simulink model "dSpaceModel_2"  (R2023a)
settings: Solver=ode1  StartTime=0.0  StopTime=inf  FixedStep=0.001  RelTol=1e-3
PostLoadFcn:
  | , if any(exist('dsrtsu_mdlpostloadfcn', 'file') ~= 0), dsrtsu_mdlpostloadfcn('Execute', bdroot); end,
InitFcn:
  | , if any(exist('rtifpga_mdlclblib', 'file') ~= 0), rtifpga_mdlclblib('Init', bdroot); end,
model workspace (MAT data in the model file):
  mode = 2
libraries: rti1202serlib x5, simulink x2, svdutilitieslib x1
(part 1 of 3)
Description:
  | Standard RTI1202 template.
  | Supported MATLAB version:  R2023a.
settings Model: Tag=RTI1202  DSRTSU_INTERNAL_RTI_VER=620  DSRTSU_INTERNAL_RTI_TYPE=rti1202  RTICANMMDATA=struct('GeneralSetupData',struct('modelroot','C:\Users\VM-User\Desktop\MigrationScripts','generalsettings',struct('filesettings',struct('destfolder',struct('Name','RTICANMM_FILES','Check',1),'buildfolder',struct('Name','.','Check',1),'AbsDestfolder',struct('Name','C:\Users\VM-User\Desktop\MigrationScripts\RTICANMM_FILES'),'AbsBuildfolder',struct('Name','C:\Users\VM-User\Desktop\MigrationScripts'))),'options',struct('addpaths',1,'rmpaths',1,'addtrcexclusion',true,'cannavigator',struct('checkmonitoring',0),'show_usrtrc',0,'use_usrtrc',0),'advanced',struct('options',ones(1,100)),'MPSetup',{{}},'RTI',struct('Type','RTI1202','Ver','7.17','Date','02-Nov-2021'),'modelname','','block','untitled'))  DSRTSU_INTERNAL_RTIFPGA=200  DSRTSU_INTERNAL_RTISTBM_VER=23.1  Creator=yd12yqyf  LastModifiedBy=ej62ixyv
settings SolverCC: AlgebraicLoopSolver=TrustRegion
settings DataIOCC: ReturnWorkspaceOutputs=off
settings OptimizationCC: BlockReduction=off  OptimizeBlockIOStorage=off  BufferReuse=off  ReuseModelBlockBuffer=off  GlobalBufferReuse=off  ExpressionFolding=off  LocalBlockOutputs=off  OptimizeDataStoreBuffers=off  BusAssignmentInplaceUpdate=off
settings DebuggingCC: UnderSpecifiedDataTypeMsg=warning  UnconnectedInputMsg=warning  UnconnectedOutputMsg=warning  UnconnectedLineMsg=warning  PregeneratedLibrarySubsystemCodeDiagnostic=none  UnderSpecifiedDimensionMsg=warning  ArithmeticOperatorsInVariantConditions=warning
settings HardwareCC: ProdBitPerPointer=32  ProdBitPerSizeT=32  ProdBitPerPtrDiffT=32  ProdLargestAtomicInteger=Integer  ProdEndianess=BigEndian  ProdWordSize=32  ProdLongLongMode=on  ProdHWDeviceType=Custom Processor->Custom  TargetIntDivRoundTo=Zero  TargetEndianess=BigEndian  TargetHWDeviceType=Custom Processor->Custom
settings ModelReferenceCC: EnableRefExpFcnMdlSchedulingChecks=on  EnableParallelModelReferenceBuilds=on  ParallelModelReferenceMATLABWorkerInit=Load Top Model
settings SFSimCC: SimUseLocalCustomCode=off  MATLABDynamicMemAlloc=off  CustomCodeUndefinedFunction=UseInterfaceOnly
settings RTWCC: Description=dSPACE DS1202 Hardware Platform  SystemTargetFile=rti1202.tlc  MakeCommand=make_rti  TemplateMakefile=rti1202.tmf  RTWUseLocalCustomCode=off  DLArmComputeVersion=19.05
settings CodeAppCC: StateflowObjectComments=on
settings STFCustomTargetCC: ParMdlRefBuildCompliant=on  ConcurrentExecutionCompliant=off  GRTInterface=off  UseToolchainInfoCompliant=off  SystemTargetFile=rti1202.tlc
settings GRTTargetCC: CompOptLevelCompliant=off  ConcurrentExecutionCompliant=off  CombineOutputUpdateFcns=off  MatFileLogging=off  CPPClassGenCompliant=off  UseToolchainInfoCompliant=off
settings ConfigComp: CovMetricSettings=dswe

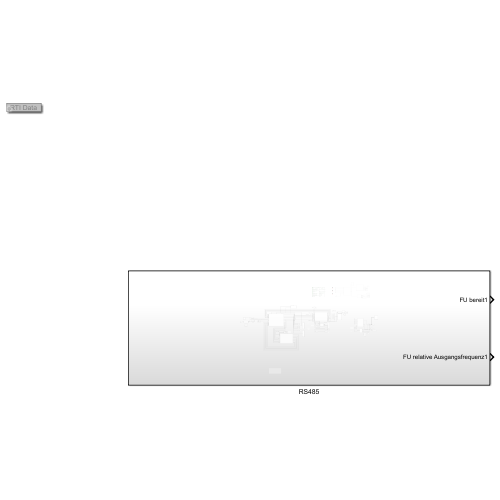
[thumbnail: Simulink's stored preview of the top-level diagram]
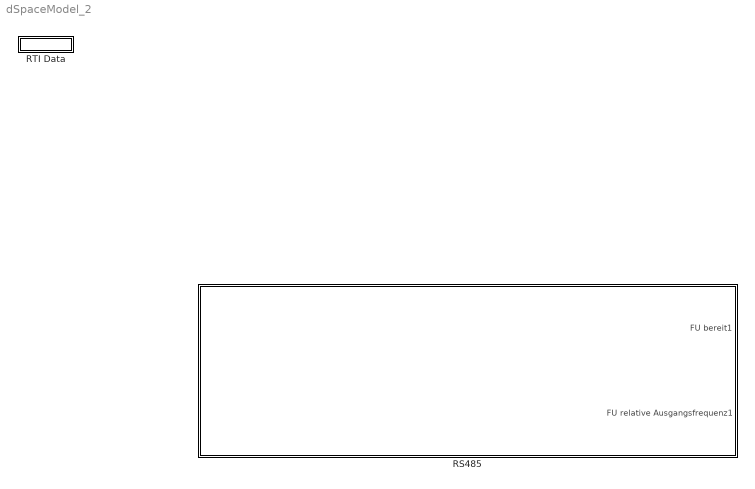
== system dSpaceModel_2 ==
  RS485 : Subsystem
  RTI Data : Subsystem  Tag=struct('RTIDataServer',struct('RTIDataServerVs','2','RTIModelDescription','struct(''main'',''dSpaceModel_2'',''sub'',''dSpaceModel_2'',''isMp'',0)'))  LoadFcn="if exist('rtidc'), try,  rtidc('DataHostBlockClbLoad', gcbh); catch, disp(['Warning: ''LoadFcn'' for RTI Data block failed: ' lasterr]); end, end,"  mask(RTI_DATA_HOST){}
      mask help:
      | RTI Data Block.
      | This block is used by RTI to store internal model-dependent data.
      | Please keep this block on the root level of the model. Deleting this block will result in data loss.
      |
      | NEVER DELETE OR COPY THIS BLOCK!
      settings: CopyFcn="if exist('rtidc'), try,  rtidc('DataHostBlockClbCopy', gcbh); catch, disp(['Warning: ''CopyFcn'' for RTI Data block failed: ' lasterr]); end, end,"  DeleteFcn="if exist('rtidc'), try,  rtidc('DataHostBlockClbDelete', gcbh); catch, disp(['Warning: ''DeleteFcn'' for RTI Data block failed: ' lasterr]); end, end,"  ModelCloseFcn="if exist('rtidc'), try,  rtidc('DataHostBlockClbModelClose', gcbh); catch, disp(['Warning: ''ModelCloseFcn'' for RTI Data block failed: ' lasterr]); end, end,"  PreSaveFcn="if exist('rtidc'), try,  rtidc('DataHostBlockClbPreSave', gcbh); catch, disp(['Warning: ''PreSaveFcn'' for RTI Data block failed: ' lasterr]); end, end,"  PostSaveFcn="if exist('rtidc'), try,  rtidc('DataHostBlockClbPostSave', gcbh); catch, disp(['Warning: ''PostSaveFcn'' for RTI Data block failed: ' lasterr]); end, end,"  NameChangeFcn="if exist('rtidc'), try,  rtidc('DataHostBlockClbNameChange', gcbh); catch, disp(['Warning: ''NameChangeFcn'' for RTI Data block failed: ' lasterr]); end, end,"
      mask Help:
      | RTI Data Block.
      | This block is used by RTI to store internal model-dependent data.
      | Please keep this block on the root level of the model. Deleting this block will result in data loss.
      | 
      | NEVER DELETE OR COPY THIS BLOCK!
      mask Display:
      | text(0.5, 0.5, 'RTI Data', 'HorizontalAlignment', 'center');
      | plot([1 0]);

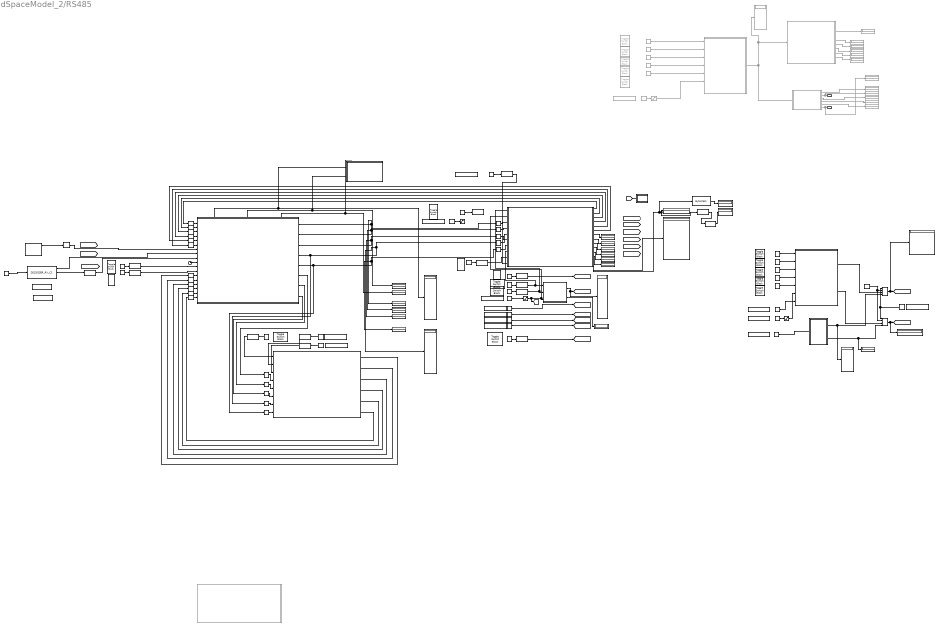
== system dSpaceModel_2/RS485 ==
  note: RX_Data
  note: THRE
  note: %| Bit| Bit value = 0 | Bit value = 1 |
      | %|----|--------------------------------------|------------------------------------|
      | %| 00 | selection between the four "3-10 Preset reference [0]...[3]" |
      | %| 01 | --""-- |
      | %|----|--------------------------------------|------------------------------------|
      | %| 02 | DC brake and stop | performs ramp |
      | %|----|--------------------------------------|------------------------------------|
      | %| 03 | lets the motor coast | starts the motor if conditions are met |
      | %|----|--------------------------------------|------------------------------------|
      | %| 04 | motor speed decreases until stop | |
      | %|----|--------------------------------------|------------------------------------|
      | %| 05 | current output frequency is stored | |
      | %|----|--------------------------------------|------------------------------------|
      | %| 06 | stop using ramp time | starts the motor if conditions are met |
      | %|----|--------------------------------------|------------------------------------|
      | %| 07 | no reset | reset |
      | %|----|--------------------------------------|------------------------------------|
      | %| 08 | | output frequency "3-19 Jog [RPM]" |
      | %|----|--------------------------------------|------------------------------------|
      | %| 09 | ramp 1 active ("3-41" and "3-42") | ramp 2 active ("3-51" and "3-52") |
      | %|----|--------------------------------------|------------------------------------|
      | %| 10 | control word is ignored | control word is used |
      | %|----|--------------------------------------|------------------------------------|
      | %| 11 | relay 01 not activated | relay 01 activated |
      | %|----|--------------------------------------|------------------------------------|
      | %| 12 | relay 04 not activated | relay 04 activated |
      | %|----|--------------------------------------|------------------------------------|
      | %| 13 | parameter set selection "0-10" and "8-55" |
      | %| 14 | |
      | %|----|--------------------------------------|------------------------------------|
      | %| 15 | no reversal | reversal |
  note: expect_len_ZKDM
  note: expect_crc_kind_ZKDM
  note: expect_addr_ZKDM
  note: req_len
  note: req_bytes
  note: req_valid
  note: resp_len
  note: resp_data
  note: resp_err_ZKDM
  note: resp_ok_ZKDM
  note: grant_ZKDM
  note: tx data
  note: tx len
  note: tx trigger
  note: temperature
  Active : Constant  Value=0
  BUS MASTER FSM : Stateflow chart  TreatAsAtomicUnit=on
      settings: PortSchema="{\"entries\":[{\"content\":{\"sides\":[{\"content\":{\"connectorIds\":[\"In4\",\"In16\",\"In18\",\"In8\",\"In14\",\"In10\",\"In1\",\"In2\",\"In3\",\"In6\",\"In11\",\"In12\",\"In5\",\"In15\",\"In17\",\"In7\",\"In13\",\"In9\"]},\"type\":\"ConnectorPlacement.EquallySpacedRectSide\",\"uuid\":\"833d115e-8081-4cb1-98c4-083d374565ad\"},{\"content\":{\"connectorIds\":[\"Out4\",\"Out6\",\"Out5\",\"Out7\",\"Out9\",\"Out10\",\"Out11\",\"Out8\"],\"side\":\"RIGHT\"},\"type\":\"ConnectorPlacement.EquallySpacedRectSide\",\"uuid\":\"f0cbf871-5cea-4f22-8059-874c69130aa3\"},{\"content\":{\"connectorIds\":[\"Out1\",\"Out2\",\"Out3\"],\"side\":\"TOP\"},\"type\":\"ConnectorPlacement.EquallySpacedRectSide\",\"uuid\":\"9def79f2-ef8f-4b80-a903-98ac734b5ab3\"}]},\"type\":\"ConnectorPlacement.EquallySpacedConnector\",\"uuid\":\"db046b19-190e-410f-b654-5051c870f3be\"}],\"packageUris\":[\"http://schema.mathworks.com/mf0/Connector/R2020b\"],\"version\":\"1.0\"}"
  Begrenzung Arbeitstemperatur1 : Saturate  UpperLimit=100  LowerLimit=0  OutDataTypeStr=uint8
  Begrenzung Arbeitstemperatur2 : Saturate  Commented=on  UpperLimit=100  LowerLimit=0
  Begrenzung Arbeitstemperatur3 : Saturate  UpperLimit=100  LowerLimit=0
  Bit Index 6: Transmitter holding register empty (THRE) indicator1 : Selector  InputPortWidth=8  IndexOptions=Starting index (dialog)  Indices=[6]  OutputSizes=1
  Byte Pack : svdutilitieslib/Byte Pack  maskPackedDataType=uint16  datatypes={'uint8'}  byteAlign=1  blockPlatform=tic2000
      settings: LibrarySourceBlock=c2000lib/Target Communication/Byte Pack
  Cast : DataTypeConversion  OutDataTypeStr=uint8  SaturateOnIntegerOverflow=off  RndMeth=Floor
  Cast To Boolean{,1..7,9} (9 alike) : DataTypeConversion  OutDataTypeStr=boolean  SaturateOnIntegerOverflow=off  RndMeth=Floor
  Cast To Boolean10 : DataTypeConversion  OutDataTypeStr=double  SaturateOnIntegerOverflow=off  RndMeth=Floor
  Cast To Boolean11 : DataTypeConversion  OutDataTypeStr=uint8  SaturateOnIntegerOverflow=off  RndMeth=Floor
  Cast To Boolean8 : DataTypeConversion  OutDataTypeStr=double  SaturateOnIntegerOverflow=off  RndMeth=Floor
  Cast To Double : DataTypeConversion  OutDataTypeStr=double  SaturateOnIntegerOverflow=off  RndMeth=Floor
  Cast1 : DataTypeConversion  OutDataTypeStr=uint16  SaturateOnIntegerOverflow=off  RndMeth=Floor
  Clock : Clock
  Constant : Constant  Value=0
  Constant1 : Constant
  Constant10 : Constant
  Constant11 : Constant  Value=34
  Constant12 : Constant  Value=8  OutDataTypeStr=double
  Constant13 : Constant  Value=125
  Constant15 : Constant  Value=0  OutDataTypeStr=uint8
  Constant16 : Constant  Value=0
  Constant19 : Constant  Value=8  OutDataTypeStr=uint32
  Constant2 : Constant  Commented=on  Value=34
  Constant5 : Constant  Value=0
  Constant6 : Constant  Value=12  OutDataTypeStr=uint8
  Constant7 : Constant  Value=31  OutDataTypeStr=uint8
  Constant8 : Constant  Value=8  OutDataTypeStr=uint8
  ConstantSwitch{1,3..6} (5 alike) : Constant  Commented=on
  ConstantSwitch{2,8..11,14} (6 alike) : Constant  Value=0
  ConstantSwitch12 : Constant  Value=34
  ConstantSwitch13 : Constant  Value=10
  ConstantSwitch7 : Constant
  Create 8-Bytes Command : MATLAB Function  TreatAsAtomicUnit=on
  DS1202SER_RX_C2 : rti1202serlib/DS1202SER_RX_C1  Reserved1=[]  Reserved2=[]  Reserved3=[]  Reserved4=[]  DSProperties=struct('RTI',struct('IOBoardType',{{'DS1202','SER'}},'SlaveProcessor','NONE','Version',uint32(1),'BlockType',struct('isSLSource',uint8(1),'isSLSink',uint8(1),'isHWSource',uint8(0),'isHWSink',uint8(1),'isSetup',uint8(0),'isInline',uint8(1),'isNonInline',uint8(0),'isInterrupt',uint8(0),'isChannelwise',uint8(1)),'UnitType','GENSER','Identifier','RECEIVE','DialogType','ML','BlockSet','NONE'))  RTIBlockInterface=struct('BlockName',struct('Token',{{'DS1202SER_RX_C'}},'BlockParam',{{'ChannelNo'}}),'InputPortsWidth',int32(1),'InputPortsActive',1,'InputPortsDataType',{{'SS_UINT32'}},'InputPortsName',{{'NumBytes'}},'OutputPortsWidth',int32([127 1 1]),'OutputPortsActive',[1 1 1],'OutputPortsDataType',{{'SS_UINT8','SS_UINT32','SS_INT32'}},'OutputPortsName',{{'RXBytes','NumRXBytes','Status'}},'BlockDisplay',{{['Serial Receive'],'center'}},'IconTransparency','on','ParameterTunableNames',{{'BytesRefNumOf'}},'InitLevel',2,'DialogFcn','guigenserreceive','MaskDescription',['To read data from the UART SW FIFO.'])  RTIBlockParameters=struct('BoardNo',{{1,'ON',[1 1]}},'ChannelNo',{{2,'ON',[1 2]}},'ChannelNumOf',{{2,'OFF',[]}},'ReceptionDataMode',{{2,'OFF',[]}},'ParamTunableMode',{{1,'OFF',[]}},'BytesRefNumOfT',{{'1','OFF',[1 inf]}},'BytesRefNumOfNT',{{'1','OFF',[1 inf]}},'BytesRefNumOfMax',{{'127','OFF',[1 inf]}},'BytesRefNumOfMode',{{0,'OFF',[]}},'BytesActNumOfMode',{{1,'OFF',[]}},'ReceptionStatusMode',{{1,'OFF',[]}},'FifoSizeDefault',{{64,'OFF',[]}},'TLCFileName',{{'rtigenserreceive','OFF',[]}})  RTISFcnParameters=struct('BoardNo','double','ChannelNo','double','ChannelNumOf','double','ReceptionDataMode','double','ParamTunableMode','double','BytesRefNumOfT','double','BytesRefNumOfNT','double','BytesRefNumOfMax','double','BytesRefNumOfMode','double','BytesActNumOfMode','double','ReceptionStatusMode','double','TLCFileName','char')  RTIBlockParaDefault=struct('BoardNo',1,'ChannelNo',1,'ChannelNumOf',2,'ReceptionDataMode',1,'ParamTunableMode',1,'BytesRefNumOfT',1,'BytesRefNumOfNT',1,'BytesRefNumOfMax',1,'BytesRefNumOfMode',0,'BytesActNumOfMode',1,'ReceptionStatusMode',1,'FifoSizeDefault',64,'TLCFileName','rtigenserreceive')
  DS1202SER_SETUP_C1 : rti1202serlib/DS1202SER_SETUP_C1  Reserved1=[]  Reserved2=[]  Reserved3=[]  Reserved4=[]  DSProperties=struct('RTI',struct('Version',uint32(2),'IOBoardType',{{'DS1202','SER'}},'SlaveProcessor','NONE','BlockType',struct('isSLSource',uint8(0),'isSLSink',uint8(0),'isHWSource',uint8(0),'isHWSink',uint8(0),'isSetup',uint8(1),'isInline',uint8(1),'isNonInline',uint8(0),'isInterrupt',uint8(0),'isChannelwise',uint8(1)),'UnitType','GENSER','Identifier','SETUP','DialogType','ML','BlockSet','NONE'))  RTIBlockInterface=struct('BlockName',struct('Token',{{'DS1202SER_SETUP_C'}},'BlockParam',{{'ChannelNo'}}),'BlockDisplay',{{['Serial Setup'],'center'}},'IconTransparency','off','ParameterTunableNames',{{}},'InitLevel',1,'DialogFcn','guigensersetup','MaskDescription',['To set the global specifications for the UART interface.'])  RTIBlockParameters=struct('ParityMode',{{3,'OFF',[1 5]}},'TransceiverMode',{{[3;1],'OFF',[]}},'QuartzFrequency',{{'160000000','OFF',[]}},'BoardNo',{{1,'ON',[1 1]}},'ChannelNo',{{1,'ON',[1 2]}},'ChannelNumOf',{{2,'OFF',[]}},'BaudRate',{{'9600','OFF',[]}},'DataBitsNumOf',{{4,'OFF',[1 4]}},'StopBitsNumOf',{{1,'OFF',[1 3]}},'ReceiveIntLevelUart',{{1,'OFF',[1 4]}},'AutoflowMode',{{0,'OFF',[]}},'FifoSize',{{'128','OFF',[]}},'ReceiveIntLevelFifo',{{0,'OFF',[]}},'FifoOverrunMode',{{1,'OFF',[]}},'FifoBlockSize',{{'0','OFF',[]}},'TermMode',{{1,'OFF',[]}},'TLCFileName',{{'rtigensersetup','OFF',[]}})  RTISFcnParameters=struct('BoardNo','double','ChannelNo','double','ChannelNumOf','double','BaudRate','double','DataBitsNumOf','double','StopBitsNumOf','double','ParityMode','double','TransceiverMode','double','ReceiveIntLevelUart','double','AutoflowMode','double','FifoSize','double','ReceiveIntLevelFifo','double','FifoBlockSize','double','TermMode','double','QuartzFrequency','double','TLCFileName','char')  RTIBlockParaDefault=struct('ParityMode',1,'TransceiverMode',[1;1],'QuartzFrequency',160000000,'BoardNo',1,'ChannelNo',1,'ChannelNumOf',2,'BaudRate',115200,'DataBitsNumOf',4,'StopBitsNumOf',1,'ReceiveIntLevelUart',4,'AutoflowMode',0,'FifoSize',64,'ReceiveIntLevelFifo',0,'FifoOverrunMode',1,'FifoBlockSize',0,'TermMode',1,'TLCFileName','rtigensersetup')
  DS1202SER_SETUP_C2 : rti1202serlib/DS1202SER_SETUP_C1  Reserved1=[]  Reserved2=[]  Reserved3=[]  Reserved4=[]  DSProperties=struct('RTI',struct('Version',uint32(2),'IOBoardType',{{'DS1202','SER'}},'SlaveProcessor','NONE','BlockType',struct('isSLSource',uint8(0),'isSLSink',uint8(0),'isHWSource',uint8(0),'isHWSink',uint8(0),'isSetup',uint8(1),'isInline',uint8(1),'isNonInline',uint8(0),'isInterrupt',uint8(0),'isChannelwise',uint8(1)),'UnitType','GENSER','Identifier','SETUP','DialogType','ML','BlockSet','NONE'))  RTIBlockInterface=struct('BlockName',struct('Token',{{'DS1202SER_SETUP_C'}},'BlockParam',{{'ChannelNo'}}),'BlockDisplay',{{['Serial Setup'],'center'}},'IconTransparency','off','ParameterTunableNames',{{}},'InitLevel',1,'DialogFcn','guigensersetup','MaskDescription',['To set the global specifications for the UART interface.'])  RTIBlockParameters=struct('ParityMode',{{3,'OFF',[1 5]}},'TransceiverMode',{{[3;3],'OFF',[]}},'QuartzFrequency',{{'160000000','OFF',[]}},'BoardNo',{{1,'ON',[1 1]}},'ChannelNo',{{2,'ON',[1 2]}},'ChannelNumOf',{{2,'OFF',[]}},'BaudRate',{{'9600','OFF',[]}},'DataBitsNumOf',{{3,'OFF',[1 4]}},'StopBitsNumOf',{{1,'OFF',[1 3]}},'ReceiveIntLevelUart',{{1,'OFF',[1 4]}},'AutoflowMode',{{0,'OFF',[]}},'FifoSize',{{'128','OFF',[]}},'ReceiveIntLevelFifo',{{0,'OFF',[]}},'FifoOverrunMode',{{1,'OFF',[]}},'FifoBlockSize',{{'0','OFF',[]}},'TermMode',{{1,'OFF',[]}},'TLCFileName',{{'rtigensersetup','OFF',[]}})  RTISFcnParameters=struct('BoardNo','double','ChannelNo','double','ChannelNumOf','double','BaudRate','double','DataBitsNumOf','double','StopBitsNumOf','double','ParityMode','double','TransceiverMode','double','ReceiveIntLevelUart','double','AutoflowMode','double','FifoSize','double','ReceiveIntLevelFifo','double','FifoBlockSize','double','TermMode','double','QuartzFrequency','double','TLCFileName','char')  RTIBlockParaDefault=struct('ParityMode',1,'TransceiverMode',[1;1],'QuartzFrequency',160000000,'BoardNo',1,'ChannelNo',1,'ChannelNumOf',2,'BaudRate',115200,'DataBitsNumOf',4,'StopBitsNumOf',1,'ReceiveIntLevelUart',4,'AutoflowMode',0,'FifoSize',64,'ReceiveIntLevelFifo',0,'FifoOverrunMode',1,'FifoBlockSize',0,'TermMode',1,'TLCFileName','rtigensersetup')
  DS1202SER_STAT_C1 : rti1202serlib/DS1202SER_STAT_C1  Reserved1=[]  Reserved2=[]  Reserved3=[]  Reserved4=[]  DSProperties=struct('RTI',struct('IOBoardType',{{'DS1202','SER'}},'SlaveProcessor','NONE','Version',uint32(1),'BlockType',struct('isSLSource',uint8(1),'isSLSink',uint8(0),'isHWSource',uint8(0),'isHWSink',uint8(0),'isSetup',uint8(0),'isInline',uint8(1),'isNonInline',uint8(0),'isInterrupt',uint8(0),'isChannelwise',uint8(1)),'UnitType','GENSER','Identifier','STATUS','DialogType','ML','BlockSet','NONE'))  RTIBlockInterface=struct('BlockName',struct('Token',{{'DS1202SER_STAT_C'}},'BlockParam',{{'ChannelNo'}}),'OutputPortsWidth',int32([8 8 8]),'OutputPortsActive',[1 1 1],'OutputPortsName',{{'Line','Modem','Interrupt'}},'OutputPortsDataType',{{'SS_BOOLEAN','SS_BOOLEAN','SS_BOOLEAN'}},'BlockDisplay',{{['Serial Status'],'left'}},'IconTransparency','on','ParameterTunableNames',{{}},'InitLevel',1,'DialogFcn','guigenserstatus','MaskDescription',['To read the contents of the UART status register.'])  RTIBlockParameters=struct('BoardNo',{{1,'ON',[1 1]}},'ChannelNo',{{1,'ON',[1 2]}},'ChannelNumOf',{{2,'OFF',[]}},'LineStatUartMode',{{1,'OFF',[]}},'ModemStatUartMode',{{1,'OFF',[]}},'InterruptStatUartMode',{{1,'OFF',[]}},'TLCFileName',{{'rtigenserstatus','OFF',[]}})  RTISFcnParameters=struct('BoardNo','double','ChannelNo','double','ChannelNumOf','double','LineStatUartMode','double','ModemStatUartMode','double','InterruptStatUartMode','double','TLCFileName','char')  RTIBlockParaDefault=struct('BoardNo',1,'ChannelNo',1,'ChannelNumOf',2,'LineStatUartMode',1,'ModemStatUartMode',1,'InterruptStatUartMode',1,'TLCFileName','rtigenserstatus')
  Display{,1,9,16..36} (24 alike) : Display
      Display19 settings: Decimation=16
      Display21 settings: Decimation=16
      Display22 settings: Decimation=16
      Display25 settings: Decimation=8
      Display30 settings: Format=binary (Stored Integer)  Decimation=8
      Display31 settings: Format=binary (Stored Integer)
      Display32 settings: Format=decimal (Stored Integer)
  Display{2..8,10..15} (13 alike) : Display  Commented=on
      Display15 settings: Decimation=8
  Edit{,1,3..13} (13 alike) : EditField  LabelPosition=Hide  ShowInitialText=on  Alignment=Center
  Edit2 : EditField  Commented=on  LabelPosition=Hide  ShowInitialText=on  Alignment=Center
  From : From
  Goto : Goto
  Invalid CTW : Constant  Value=0
  Invalid CTW1 : Constant
  Length : Constant  Value=6  OutDataTypeStr=uint8
  MATLAB Function : MATLAB Function  TreatAsAtomicUnit=on
  MATLAB Function1 : MATLAB Function  TreatAsAtomicUnit=on
  MATLAB Function2 : MATLAB Function  Commented=on  TreatAsAtomicUnit=on
  MATLAB Function3 : MATLAB Function  Commented=on  TreatAsAtomicUnit=on
  MATLAB Function4 : MATLAB Function  TreatAsAtomicUnit=on
  Memory{,1..21} (22 alike) : Memory
  Multiport Switch : MultiPortSwitch  DataPortOrder=Zero-based contiguous  zeroidx=on  AllowDiffInputSizes=on  SaturateOnIntegerOverflow=off  InputSameDT=off
  Multiport Switch1 : MultiPortSwitch  DataPortOrder=Zero-based contiguous  zeroidx=on  SaturateOnIntegerOverflow=off  InputSameDT=off
  RX on : Constant  Value=0
  Saturation : Saturate  UpperLimit=100  LowerLimit=0
  Setpoint : Constant  Value=100
  Subsystem : Subsystem
  Subsystem2 : Subsystem  Commented=on
  THERMO FSM : Stateflow chart  TreatAsAtomicUnit=on
      settings: PortSchema="{\"entries\":[{\"content\":{\"sides\":[{\"content\":{\"connectorIds\":[\"In1\",\"In8\",\"In2\",\"In3\",\"In4\",\"In5\",\"In6\",\"In7\"]},\"type\":\"ConnectorPlacement.EquallySpacedRectSide\",\"uuid\":\"871d9cfd-145d-45d5-a3f3-b0fbfa7fca38\"},{\"content\":{\"connectorIds\":[\"Out1\",\"Out2\",\"Out3\",\"Out4\",\"Out5\",\"Out6\"],\"side\":\"RIGHT\"},\"type\":\"ConnectorPlacement.EquallySpacedRectSide\",\"uuid\":\"1294343c-a8c7-4cfc-abe5-8e317e926a90\"},{\"content\":{\"side\":\"TOP\"},\"type\":\"ConnectorPlacement.EquallySpacedRectSide\",\"uuid\":\"15bb1215-e2cd-495a-a77a-921f6d2a5d53\"}]},\"type\":\"ConnectorPlacement.EquallySpacedConnector\",\"uuid\":\"a3eba055-3d67-4b5b-8035-4f59ba25cafd\"}],\"packageUris\":[\"http://schema.mathworks.com/mf0/Connector/R2020b\"],\"version\":\"1.0\"}"
  TX on : Constant
  Toggle Switch{1..2,8..16,18..20} (14 alike) : ToggleSwitchBlock
      settings: Values={{'Off', 'On'}, [0 1]}
  Toggle Switch{3..7} (5 alike) : ToggleSwitchBlock  Commented=on
      settings: Values={{'Off', 'On'}, [0 1]}
  Variant Subsystem : Subsystem  Commented=on  Variant=on
  ZKDM FSM : Stateflow chart  TreatAsAtomicUnit=on
  FU bereit1 : Outport
  FU relative Ausgangsfrequenz1 : Outport  Port=2
  wires:
  Constant1/1 -> Begrenzung Arbeitstemperatur1/1
  Clock/1 -> BUS MASTER FSM/6(now)
  BUS MASTER FSM/4(grant_ZKDM) -> Display16/1, Memory/1
  BUS MASTER FSM/6(resp_ok_ZKDM) -> Memory1/1, Display17/1
  BUS MASTER FSM/5(resp_err_ZKDM) -> Memory2/1, Display18/1
  BUS MASTER FSM/7(resp_data) -> Display19/1, Memory3/1, Memory14/1
  BUS MASTER FSM/9(resp_len) -> Memory4/1, Display20/1, Memory15/1
  BUS MASTER FSM/1(TX_Data) -> Display22/1, Subsystem/1(TXBytes)
  BUS MASTER FSM/2(TX_Len) -> Display23/1, Subsystem/2(NumBytes)
  BUS MASTER FSM/3(TX_Trigger) -> Display24/1, Subsystem/Trigger
  ZKDM FSM/1(req_valid) -> Memory5/1
  ZKDM FSM/2(req_bytes) -> Memory6/1
  ZKDM FSM/3(req_len) -> Memory7/1
  ZKDM FSM/4(expect_addr_ZKDM) -> Memory8/1
  ZKDM FSM/6(expect_len_ZKDM) -> Memory9/1
  ZKDM FSM/5(expect_crc_kind_ZKDM) -> Memory10/1
  MATLAB Function3/1(u) -> Subsystem2/1(Antworttelegramm), Display15/1, MATLAB Function2/1(u)
  Begrenzung Arbeitstemperatur2/1 -> MATLAB Function3/6(freq_rel_percent)
  Constant2/1 -> Begrenzung Arbeitstemperatur2/1
  ConstantSwitch1/1 -> MATLAB Function3/1(fu_ctrl_ready)
  ConstantSwitch3/1 -> MATLAB Function3/2(fu_ready)
  ConstantSwitch4/1 -> MATLAB Function3/3(fault_trip)
  ConstantSwitch5/1 -> MATLAB Function3/4(fault_no_trip)
  ConstantSwitch6/1 -> MATLAB Function3/5(bus_control_active)
  MATLAB Function2/3(freq_rel_percent) -> Display2/1
  MATLAB Function2/5(fu_ctrl_ready) -> Display3/1
  MATLAB Function2/6(fu_ready) -> Display4/1
  MATLAB Function2/7(fault_trip) -> Display5/1
  MATLAB Function2/8(fault_no_trip) -> Display6/1
  MATLAB Function2/9(bus_control_active) -> Display7/1
  Subsystem2/5(Bussteuerung aktive) -> Display14/1
  Subsystem2/2(FU bereit) -> Display11/1, FU bereit1/1
  Subsystem2/1(Steuerung FU bereit) -> Display10/1
  Subsystem2/6(relative Ausgangsfrequenz) -> Display8/1, FU relative Ausgangsfrequenz1/1
  Subsystem2/3(Fehler mit Abschaltung) -> Display12/1
  Subsystem2/4(Fehler ohne Abschaltung) -> Display13/1
  Cast To Boolean/1 -> ZKDM FSM/8(invalid_flag), Create 8-Bytes Command/1(invalid_control_word)
  Cast To Boolean1/1 -> ZKDM FSM/1(active), Create 8-Bytes Command/2(active)
  Saturation/1 -> Goto/1, Create 8-Bytes Command/3(setpoint), ZKDM FSM/2(setpoint)
  Invalid CTW/1 -> Cast To Boolean/1
  Active/1 -> Cast To Boolean1/1
  Setpoint/1 -> Saturation/1
  Constant5/1 -> Cast To Boolean2/1
  Constant6/1 -> [expect_addr_ZKDM]
  Constant7/1 -> [expect_crc_kind_ZKDM]
  Constant8/1 -> [expect_len_ZKDM]
  Length/1 -> [req_len]
  Cast To Boolean2/1 -> [req_valid]
  Create 8-Bytes Command/1(command) -> Display21/1, [req_bytes]
  Cast To Boolean3/1 -> [THRE]
  Constant10/1 -> Cast To Boolean3/1
  Begrenzung Arbeitstemperatur3/1 -> MATLAB Function4/6(freq_rel_percent)
  ConstantSwitch10/1 -> MATLAB Function4/4(fault_no_trip)
  ConstantSwitch8/1 -> MATLAB Function4/2(fu_ready)
  ConstantSwitch11/1 -> MATLAB Function4/5(bus_control_active)
  Constant11/1 -> Begrenzung Arbeitstemperatur3/1
  ConstantSwitch7/1 -> MATLAB Function4/1(fu_ctrl_ready)
  MATLAB Function4/1(u) -> Multiport Switch/3
  ConstantSwitch9/1 -> MATLAB Function4/3(fault_trip)
  Constant13/1 -> MATLAB Function4/7(addr)
  Constant15/1 -> Multiport Switch1/2, Multiport Switch/2
  ConstantSwitch2/1 -> Cast To Boolean4/1
  Memory1/1 -> ZKDM FSM/4(resp_ok)
  Memory/1 -> ZKDM FSM/3(grant)
  Memory2/1 -> ZKDM FSM/6(resp_err)
  Memory3/1 -> ZKDM FSM/5(resp_data)
  Memory4/1 -> ZKDM FSM/7(resp_len)
  Memory5/1 -> BUS MASTER FSM/4(req_valid_ZKDM)
  Memory6/1 -> BUS MASTER FSM/16(req_bytes_ZKDM)
  Memory7/1 -> BUS MASTER FSM/18(req_len_ZKDM)
  Memory8/1 -> BUS MASTER FSM/8(expect_addr_ZKDM)
  Memory9/1 -> BUS MASTER FSM/14(expect_len_ZKDM)
  Memory10/1 -> BUS MASTER FSM/10(expect_crc_kind_ZKDM)
  Constant16/1 -> Cast To Boolean5/1
  Cast To Boolean5/1 -> ZKDM FSM/9(tx_trigger)
  Cast To Boolean6/1 -> BUS MASTER FSM/11(tx_switch)
  TX on/1 -> Cast To Boolean6/1
  Cast To Boolean7/1 -> BUS MASTER FSM/12(rx_switch)
  DS1202SER_STAT_C1/1 -> Bit Index 6: Transmitter holding register empty (THRE) indicator1/1
  Constant19/1 -> DS1202SER_RX_C2/1
  DS1202SER_RX_C2/2 -> Cast/1
  ZKDM FSM/7(fault_no_trip) -> Display/1
  ZKDM FSM/8(fault_trip) -> Display1/1
  ZKDM FSM/9(fu_ctrl_ready) -> Display9/1
  ZKDM FSM/10(fu_ready) -> Display26/1
  ZKDM FSM/11(bus_ctrl_active) -> Display27/1
  ZKDM FSM/12(freq_rel) -> Display28/1
  RX on/1 -> Cast To Boolean7/1
  Create 8-Bytes Command/2(pcd2) -> Display29/1
  ZKDM FSM/13(debug_command) -> Display30/1
  From/1 -> MATLAB Function/1(setpoint)
  ZKDM FSM/14(debug_pcd2) -> Byte Pack/1, Cast1/1, Display31/1
  ConstantSwitch12/1 -> Cast To Boolean8/1
  Cast To Boolean8/1 -> ZKDM FSM/10(off_set)
  Cast To Double/1 -> Display32/1
  Cast1/1 -> Cast To Double/1
  Byte Pack/1 -> Display33/1
  Cast/1 -> BUS MASTER FSM/3(RX_Len)
  Invalid CTW1/1 -> Cast To Boolean9/1
  Cast To Boolean9/1 -> THERMO FSM/1(active)
  ConstantSwitch13/1 -> Cast To Boolean10/1
  Cast To Boolean10/1 -> THERMO FSM/2(setpoint)
  BUS MASTER FSM/10(grant_THERMO) -> Memory11/1
  BUS MASTER FSM/11(resp_ok_THERMO) -> Memory12/1
  BUS MASTER FSM/8(resp_err_THERMO) -> Memory13/1
  Memory11/1 -> THERMO FSM/3(grant)
  Memory12/1 -> THERMO FSM/4(resp_ok)
  Memory13/1 -> THERMO FSM/5(resp_err)
  Memory15/1 -> THERMO FSM/7(resp_len)
  Memory14/1 -> THERMO FSM/6(resp_data)
  THERMO FSM/1(req_valid) -> Memory16/1
  THERMO FSM/2(req_bytes) -> Memory19/1
  THERMO FSM/3(req_len) -> Memory18/1
  THERMO FSM/4(expect_addr) -> Memory17/1
  THERMO FSM/5(expect_len) -> Memory21/1
  THERMO FSM/6(expect_crc_kind) -> BUS MASTER FSM/9(expect_crc_kind_THERMO)
  Memory16/1 -> BUS MASTER FSM/5(req_valid_THERMO)
  Memory19/1 -> BUS MASTER FSM/15(req_bytes_THERMO)
  Memory18/1 -> BUS MASTER FSM/17(req_len_THERMO)
  Memory17/1 -> BUS MASTER FSM/7(expect_addr_THERMO)
  Memory21/1 -> BUS MASTER FSM/13(expect_len_THERMO)
  Cast To Boolean11/1 -> THERMO FSM/8(commandType)
  ConstantSwitch14/1 -> Cast To Boolean11/1
  MATLAB Function4/2(length) -> Multiport Switch1/3
  MATLAB Function1/1(telegram) -> Multiport Switch/4, Display35/1
  Multiport Switch1/1 -> Display34/1, [RX_Len]
  Multiport Switch/1 -> Display25/1, [RX_Data]
  Constant/1 -> Multiport Switch/1, Multiport Switch1/1
  Constant12/1 -> MATLAB Function1/1(temp)
  MATLAB Function1/2(telegramLen) -> Display36/1, Multiport Switch1/4
  DS1202SER_RX_C2/1 -> BUS MASTER FSM/2(RX_Data)
  Bit Index 6: Transmitter holding register empty (THRE) indicator1/1 -> BUS MASTER FSM/1(THRE)

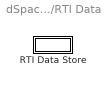
== system dSpaceModel_2/RTI Data ==
  RTI Data Store : Subsystem  Tag="struct('private',struct('version',struct('dsVer',uint32(2)),'access',struct('modified',['09-Mar-2026 11:52:44'],'type','Model','isPerm',1)),'public',struct('main',struct('data',[]),'sub',struct('name',{{'dSpaceModel_2'}},'data',{{struct('TH',struct('thTaskInfo',struct('taskType',{'TIMER','HWINT','TMRINT','SWINT','GLINT'},'tasksNumOf',{1,0,0,0,0},'srcIds',{{'TIMERA'},{},{},{},{}},'taskNames',{{['Timer Task 1']},{},{},{},{}})),'th_tc',struct('dataType','TASK','taskGroupId','','taskGroupList',{{}},'taskSchedulingPolicy','FCFS','taskType','TIMER','blkh',-1,'srcId','TIMERA','srcSgnName',['Timer A interrupt'],'srcCpuName','','taskName',['Timer Task 1  [0.001] s'],'taskNameDisplayExt','','smplTime',0.001,'smplTimeOffs',0,'hasFixedPriority',0,'priority',1,'hasFixedOvc',0,'ovcType',1,'ovcMax',1),'tc_th',struct('dataType','TASK','taskGroupId','','taskGroupList',{{}},'taskSchedulingPolicy','FCFS','taskType','TIMER','blkh',-1,'srcId','TIMERA','srcSgnName',['Timer A interrupt'],'srcCpuName','','taskName',['Timer Task 1  [0.001] s'],'taskNameDisplayExt','','smplTime',0.001,'smplTimeOffs',0,'hasFixedPriority',0,'priority',1,'hasFixedOvc',0,'ovcType',1,'ovcMax',1))}})))"  mask(RTI_DATA_STORE){}
      mask help:
      | RTI Data Store Block. This block is used by RTI to store internal model dependent data. Deleting this block will result in data loss.
      |
      | NEVER DELETE, COPY, OR MODIFY THIS BLOCK!
      mask Help:
      | RTI Data Store Block. This block is used by RTI to store internal model dependent data. Deleting this block will result in data loss.
      | 
      | NEVER DELETE, COPY, OR MODIFY THIS BLOCK!
      mask Display: text(0.5, 0.5, ' ', 'HorizontalAlignment', 'center');

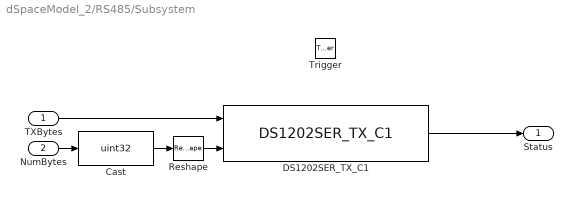
== system dSpaceModel_2/RS485/Subsystem ==
  TXBytes : Inport
  NumBytes : Inport  Port=2
  Trigger : TriggerPort  VariantControl=(inherit)  PortDimensions=1
  Cast : DataTypeConversion  OutDataTypeStr=uint32  SaturateOnIntegerOverflow=off  RndMeth=Floor
  DS1202SER_TX_C1 : rti1202serlib/DS1202SER_TX_C1  Reserved1=[]  Reserved2=[]  Reserved3=[]  Reserved4=[]  DSProperties=struct('RTI',struct('IOBoardType',{{'DS1202','SER'}},'SlaveProcessor','NONE','Version',uint32(1),'BlockType',struct('isSLSource',uint8(1),'isSLSink',uint8(1),'isHWSource',uint8(1),'isHWSink',uint8(0),'isSetup',uint8(0),'isInline',uint8(1),'isNonInline',uint8(0),'isInterrupt',uint8(0),'isChannelwise',uint8(1)),'UnitType','GENSER','Identifier','TRANSMIT','DialogType','ML','BlockSet','NONE'))  RTIBlockInterface=struct('BlockName',struct('Token',{{'DS1202SER_TX_C'}},'BlockParam',{{'ChannelNo'}}),'InputPortsWidth',int32([127 1]),'InputPortsActive',[1 1],'InputPortsDataType',{{'SS_UINT8','SS_UINT32'}},'InputPortsName',{{'TXBytes','NumBytes'}},'OutputPortsWidth',int32([1 1]),'OutputPortsActive',[0 1],'OutputPortsDataType',{{'SS_UINT32','SS_INT32'}},'OutputPortsName',{{'NumTXBytes','Status'}},'BlockDisplay',{{['Serial Transmit'],'center'}},'IconTransparency','on','ParameterTunableNames',{{'BytesRefNumOf'}},'InitLevel',2,'DialogFcn','guigensertransmit','MaskDescription',['To write data to the UART SW FIFO.'])  RTIBlockParameters=struct('BoardNo',{{1,'ON',[1 1]}},'ChannelNo',{{1,'ON',[1 2]}},'ChannelNumOf',{{2,'OFF',[]}},'TransmitFifoOverrunMode',{{1,'OFF',[]}},'ParamTunableMode',{{1,'OFF',[]}},'BytesRefNumOfT',{{'32','OFF',[1 inf]}},'BytesRefNumOfNT',{{'64','OFF',[1 inf]}},'BytesRefNumOfMax',{{'127','OFF',[1 inf]}},'BytesRefNumOfMode',{{0,'OFF',[]}},'BytesActNumOfMode',{{0,'OFF',[]}},'TransmissionStatusMode',{{1,'OFF',[]}},'FifoSizeDefault',{{64,'OFF',[]}},'TLCFileName',{{'rtigensertransmit','OFF',[]}})  RTISFcnParameters=struct('BoardNo','double','ChannelNo','double','ChannelNumOf','double','TransmitFifoOverrunMode','double','ParamTunableMode','double','BytesRefNumOfT','double','BytesRefNumOfNT','double','BytesRefNumOfMax','double','BytesRefNumOfMode','double','BytesActNumOfMode','double','TransmissionStatusMode','double','TLCFileName','char')  RTIBlockParaDefault=struct('BoardNo',1,'ChannelNo',1,'ChannelNumOf',2,'TransmitFifoOverrunMode',1,'ParamTunableMode',1,'BytesRefNumOfT',1,'BytesRefNumOfNT',1,'BytesRefNumOfMax',1,'BytesRefNumOfMode',0,'BytesActNumOfMode',1,'TransmissionStatusMode',1,'FifoSizeDefault',64,'TLCFileName','rtigensertransmit')
  Reshape : Reshape
  Status : Outport
  wires:
  TXBytes/1 -> DS1202SER_TX_C1/1
  DS1202SER_TX_C1/1 -> Status/1
  NumBytes/1 -> Cast/1
  Cast/1 -> Reshape/1
  Reshape/1 -> DS1202SER_TX_C1/2

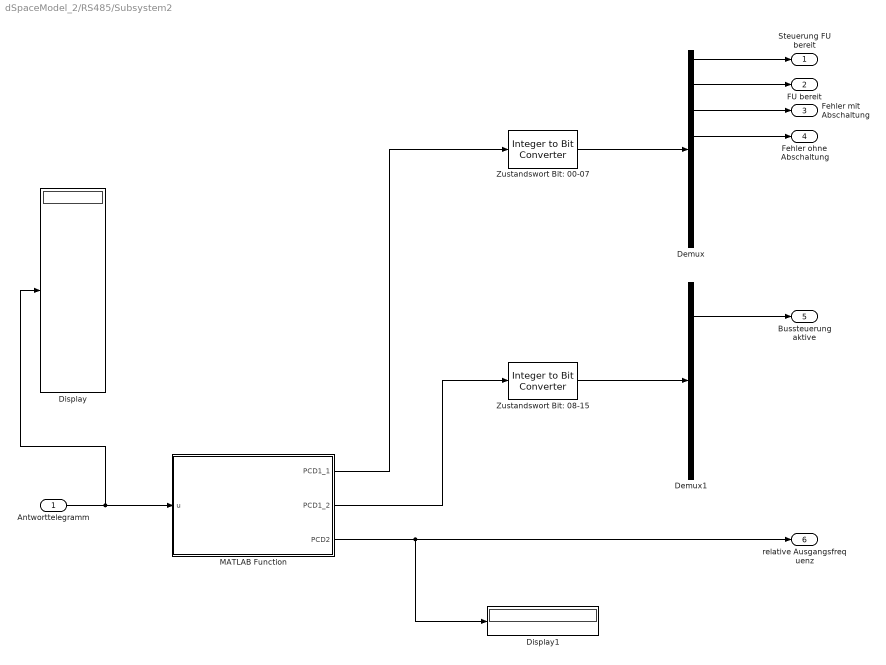
== system dSpaceModel_2/RS485/Subsystem2 ==
  Antworttelegramm : Inport
  Demux : Demux  Outputs=8
  Demux1 : Demux  Outputs=8
  Display : Display
      settings: Decimation=8
  Display1 : Display
  MATLAB Function : MATLAB Function  TreatAsAtomicUnit=on
  Zustandswort Bit: 00-07 : simulink/Logic and Bit Operations/Integer to Bit Converter  nbits=8  signedInputValues=Unsigned  bitOrder=MSB first  outDtype=boolean
  Zustandswort Bit: 08-15 : simulink/Logic and Bit Operations/Integer to Bit Converter  nbits=8  signedInputValues=Unsigned  bitOrder=MSB first  outDtype=boolean
  Steuerung FU bereit : Outport
  FU bereit : Outport  Port=2
  Fehler mit Abschaltung : Outport  Port=3
  Fehler ohne Abschaltung : Outport  Port=4
  Bussteuerung aktive : Outport  Port=5
  relative Ausgangsfrequenz : Outport  Port=6
  wires:
  MATLAB Function/3(PCD2) -> Display1/1, relative Ausgangsfrequenz/1
  MATLAB Function/2(PCD1_2) -> Zustandswort Bit: 08-15/1
  MATLAB Function/1(PCD1_1) -> Zustandswort Bit: 00-07/1
  Demux1/2 -> Bussteuerung aktive/1
  Zustandswort Bit: 08-15/1 -> Demux1/1
  Zustandswort Bit: 00-07/1 -> Demux/1
  Demux/4 -> Fehler ohne Abschaltung/1
  Demux/3 -> Fehler mit Abschaltung/1
  Demux/2 -> FU bereit/1
  Demux/1 -> Steuerung FU bereit/1
  Antworttelegramm/1 -> Display/1, MATLAB Function/1(u)

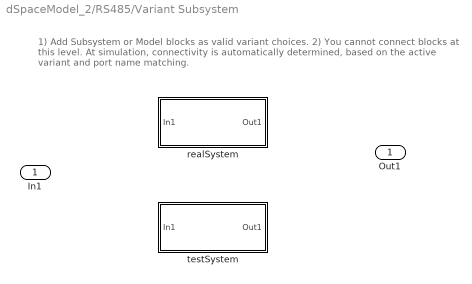
== system dSpaceModel_2/RS485/Variant Subsystem ==
  note: 1) Add Subsystem or Model blocks as valid variant choices.
      | 2) You cannot connect blocks at this level. At simulation, connectivity is automatically
      | determined, based on the active variant and port name matching.
  In1 : Inport
  realSystem : Subsystem  VariantControl=mode == 1
  testSystem : Subsystem  VariantControl=mode == 2
  Out1 : Outport

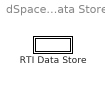
== system dSpaceModel_2/RTI Data/RTI Data Store ==
  RTI Data Store : Subsystem  mask(RTI_DATA_STORE){}
      mask help:
      | RTI Data Store Block. This block is used by RTI to store internal model dependent data. Deleting this block will result in data loss.
      |
      | NEVER DELETE, COPY, OR MODIFY THIS BLOCK!
      mask Help:
      | RTI Data Store Block. This block is used by RTI to store internal model dependent data. Deleting this block will result in data loss.
      | 
      | NEVER DELETE, COPY, OR MODIFY THIS BLOCK!
      mask Display: text(0.5, 0.5, ' ', 'HorizontalAlignment', 'center');

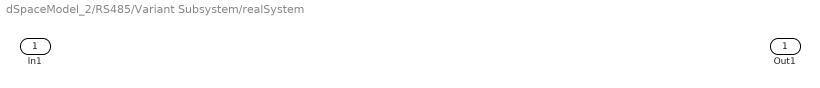
== system dSpaceModel_2/RS485/Variant Subsystem/realSystem ==
  In1 : Inport
  Out1 : Outport

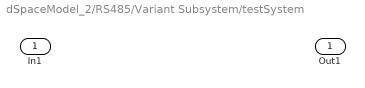
== system dSpaceModel_2/RS485/Variant Subsystem/testSystem ==
  In1 : Inport
  Out1 : Outport

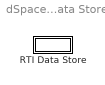
== system dSpaceModel_2/RTI Data/RTI Data Store/RTI Data Store ==
  RTI Data Store : Subsystem  mask(RTI_DATA_STORE){}
      mask help:
      | RTI Data Store Block. This block is used by RTI to store internal model dependent data. Deleting this block will result in data loss.
      |
      | NEVER DELETE, COPY, OR MODIFY THIS BLOCK!
      mask Help:
      | RTI Data Store Block. This block is used by RTI to store internal model dependent data. Deleting this block will result in data loss.
      | 
      | NEVER DELETE, COPY, OR MODIFY THIS BLOCK!
      mask Display: text(0.5, 0.5, ' ', 'HorizontalAlignment', 'center');

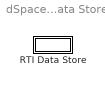
== system dSpaceModel_2/RTI Data/RTI Data Store/RTI Data Store/RTI Data Store ==
  RTI Data Store : Subsystem  mask(RTI_DATA_STORE){}
      mask help:
      | RTI Data Store Block. This block is used by RTI to store internal model dependent data. Deleting this block will result in data loss.
      |
      | NEVER DELETE, COPY, OR MODIFY THIS BLOCK!
      mask Help:
      | RTI Data Store Block. This block is used by RTI to store internal model dependent data. Deleting this block will result in data loss.
      | 
      | NEVER DELETE, COPY, OR MODIFY THIS BLOCK!
      mask Display: text(0.5, 0.5, ' ', 'HorizontalAlignment', 'center');

== system dSpaceModel_2/RTI Data/RTI Data Store/RTI Data Store/RTI Data Store/RTI Data Store ==

== matlab function dSpaceModel_2/RS485/Create 8-Bytes Command ==
  data: invalid_control_word input; active input; command output; setpoint input; pcd2 output
% Generates a telegram of the FC protocol for communication with a Danfoss frequency converter,
% telegram type: Process block (PCD) – 4 bytes
%
%##################################################################################
%Danfoss control word according to FC profile
%----------------------------------------------------------------------------------
%| Bit|                        Bit value = 0 |                     Bit value = 1  |
%|----|--------------------------------------|------------------------------------|
%| 00 | selection between the four "3-10 Preset reference [0]...[3]"             |
%| 01 | --""--                                                                   |
%|----|--------------------------------------|------------------------------------|
%| 02 |             DC brake and stop        |             performs ramp          |
%|----|--------------------------------------|------------------------------------|
%| 03 | lets the motor coast                 | starts the motor if conditions are met |
%|----|--------------------------------------|------------------------------------|
%| 04 | motor speed decreases until stop     |                                    |
%|----|--------------------------------------|------------------------------------|
%| 05 | current output frequency is stored   |                                    |
%|----|--------------------------------------|------------------------------------|
%| 06 | stop using ramp time                 | starts the motor if conditions are met |
%|----|--------------------------------------|------------------------------------|
%| 07 | no reset                             | reset                              |
%|----|--------------------------------------|------------------------------------|
%| 08 |                                      | output frequency "3-19 Jog [RPM]"  |
%|----|--------------------------------------|------------------------------------|
%| 09 | ramp 1 active ("3-41" and "3-42")    | ramp 2 active ("3-51" and "3-52")  |
%|----|--------------------------------------|------------------------------------|
%| 10 | control word is ignored              | control word is used               |
%|----|--------------------------------------|------------------------------------|
%| 11 | relay 01 not activated               | relay 01 activated                 |
%|----|--------------------------------------|------------------------------------|
%| 12 | relay 04 not activated               | relay 04 activated                 |
%|----|--------------------------------------|------------------------------------|
%| 13 | parameter set selection "0-10" and "8-55"                                |
%| 14 |                                                                            |
%|----|--------------------------------------|------------------------------------|
%| 15 | no reversal                          | reversal                           |
%----------------------------------------------------------------------------------
%##################################################################################

function [command, pcd2] = fcn(invalid_control_word, active, setpoint)

if setpoint < 0
        error('setpoint must be non-negative.');
end

command = zeros(1, 127, 'uint8');
startzeichen = uint8(2);    % Start character (STX)
telegrammlaenge = uint8(6); % Specifies telegram length: 6 or 14 data bytes (data bytes + address byte + checksum)
adresse = 0b01111101;       % Address 125 in binary, address of the frequency converter (FU)
                            % Address format 1–126 => Bit 7 = 1; FU address “10” => Bit 0–6
pcd1_1 = 0b00000100;        % Control word (CTW) bits 15 to 08
pcd1_2 = 0b00100100;        % Control word (CTW) bits 07 to 00 ... before change: 0b00101110;
bcc = 0;                    % Data control byte, Block Check Character (BCC)

% modify the flag
if (invalid_control_word == false)
    pcd1_1 = bitor(pcd1_1, 0b00100000); 
    % If invalid_flag is `false`, the result will change `pcd11` to `0b00100000`, indicating that the control word is now in use.
end

if (active == true)
    pcd1_2 = bitor(pcd1_2, 0b01111100); % set 02, 03, 04, 05, 06 to 1
    pcd1_1 = bitor(pcd1_1, 0b00000100); % Starts the motor; "0": the frequency converter lets the motor coast
end

%%- `command(4) = pcd1_1;`
  % - Value: This byte is constructed based on the input conditions (`steuerwort_invalid` and `aktiv`).
  % - It starts with `0b00000000` (initial value) and may have bits set:
  %   - Bit 5 is set to 1 if `steuerwort_invalid` is false (valid control word).
  %   - Bit 4 is set to 1 if `aktiv` is true (start command).
  % - As a result, if `aktiv` is true, the value changes:
  %     - From: `0b00100000`
  %     - To:   `0b00110000` (decimal 48), indicating that the motor should start.

% scale the speed setpoint
% Example: convert 50% speed to 16-bit integer
% 50% = (16384 / 100 * 50) = 8192
% 8192 = 0b1000000000000000 (binary)

soll = setpoint * (16384 / 100);
pcd2 = uint16(round(soll));
pcd2split = typecast(pcd2, 'uint8');

pcd2binary = dec2bin(pcd2, 16);
pcd2binaryFlipped = flip(pcd2binary);
pcd2flipped = bin2dec(pcd2binary);
%pcd2splitflipped = typecast(pcd2flipped, 'uint8');
%This is a 16-bit integer converted to two bytes that represents the desired speed (drehzahl_Sollwert) scaled to a proper range.
   %- The speed is scaled by multiplying the `drehzahl_Sollwert` by `(16384 / 100)`, allowing for a representation of the speed setting as a 16-bit integer.
   %- This is then converted from an `int16` to `uint8`, giving two bytes: `pcd2(1)` and `pcd2(2)`, with the bytes being flipped to match byte order expectations.

bcc = bitxor(startzeichen, telegrammlaenge);
bcc = bitxor(bcc, adresse);
bcc = bitxor(bcc, pcd1_1);
bcc = bitxor(bcc, pcd1_2);
bcc = bitxor(bcc, pcd2split(1));
bcc = bitxor(bcc, pcd2split(2));

command(1) = startzeichen;
command(2) = telegrammlaenge;
command(3) = adresse;
command(4) = pcd1_1; %This byte functions as part of the control command to the motor, determining how it should behave.
command(5) = pcd1_2; %This byte also forms part of the control command. It usually contains predefined flags or control commands as per the motor's specification.
command(6:7) = [bin2dec(pcd2binaryFlipped(1:8)), bin2dec(pcd2binaryFlipped(9:16))]; %This part of the command specifies the desired speed for the motor. from the user sollwert.
command(8) = bcc;

%example message:

%Address: 118 Motor Activation Flag: True Target Speed: 89% BCC is valid
%2 6 118 48 46 56 246 162
end

== matlab function dSpaceModel_2/RS485/MATLAB Function4 ==
  data: fu_ctrl_ready input; u output; fu_ready input; fault_trip input; fault_no_trip input; bus_control_active input; freq_rel_percent input; addr input; length output
function [u, length] = build_fc_rx_telegram(fu_ctrl_ready, fu_ready, fault_trip, fault_no_trip, bus_control_active, freq_rel_percent, addr)
%#codegen
% Build an 8-byte Danfoss FC "reply" telegram:
%   [STX, LEN, ADDR, STW_HI, STW_LO, OUT_HI, OUT_LO, BCC]
%
% Inputs:
%   fu_ctrl_ready       : logical  % maps to STW bit 0
%   fu_ready            : logical  % maps to STW bit 1
%   fault_trip          : logical  % maps to STW bit 2 (trip = hard fault)
%   fault_no_trip       : logical  % maps to STW bit 3 (warning)
%   bus_control_active  : logical  % maps to STW bit 12
%   freq_rel_percent    : double   % 0..100 (%) — will be clamped & rounded to Q14
%   addr                : uint8    % (optional) on-wire FC address byte; default 253
%
% Output:
%   u (1x8 uint8) = FC reply frame you can feed into your parser
%
% Notes:
% - Mapping follows the demo you showed:
%     bit0 = fu_ctrl_ready
%     bit1 = fu_ready
%     bit2 = fault_trip
%     bit3 = fault_no_trip
%     bit12 = bus_control_active
% - OUT is Q14: 0..16384 ↔ 0..100%

    if nargin < 7
        addr = uint8(253);   % default FC on-wire address (e.g., node 125)
    else
        addr = uint8(addr);
    end

    % helper: convert MSB index k (15..0) to bitset() position (1..16)
    msbpos = @(k) 16 - k;
    
    sw = uint16(0);
    if fu_ctrl_ready,      sw = bitset(sw, msbpos(0),  true); end   % bit0
    if fu_ready,           sw = bitset(sw, msbpos(1),  true); end   % bit1
    if fault_trip,         sw = bitset(sw, msbpos(2),  true); end   % bit2
    if fault_no_trip,      sw = bitset(sw, msbpos(3),  true); end   % bit3
    if bus_control_active, sw = bitset(sw, msbpos(9),  true); end   % bit9

    STW_HI = uint8(bitshift(sw, -8));
    STW_LO = uint8(bitand(sw, 255));

    % ---------- OUT (Q14) from percent ----------
    if ~isfinite(freq_rel_percent), freq_rel_percent = 0; end
    freq_rel_percent = max(0, min(100, freq_rel_percent));
    q14 = uint16(round(freq_rel_percent * (16384/100)));
    OUT_HI = uint8(bitshift(q14, -8));
    OUT_LO = uint8(bitand(q14, 255));

    % ---------- assemble frame ----------
    STX = uint8(2);
    LEN = uint8(6);   % addr + 4 data bytes + BCC

    u = zeros(1,127,'uint8');
    u(1) = STX;
    u(2) = LEN;
    u(3) = addr;
    u(4) = STW_HI;
    u(5) = STW_LO;
    u(6) = OUT_HI;
    u(7) = OUT_LO;

    % ---------- BCC (XOR of bytes 1..7) ----------
    bcc = uint8(0);
    for k = 1:7
        bcc = bitxor(bcc, u(k));
    end
    u(8) = bcc;

    length = uint8(8);
end

== matlab function dSpaceModel_2/RS485/MATLAB Function1 ==
  data: temp input size=1; telegram output; telegramLen output size=1
function [telegram, telegramLen] = thermo_telegram_u8(temp)
    %#codegen
    % Builds: 'A005_-55.5' as ASCII bytes (uint8 buffer + uint8 length)
    
    MAX = uint8(32);
    telegram = zeros(1, double(MAX), 'uint8');   % buffer is uint8; size needs double in MATLAB syntax
    telegramLen = uint8(0);
    
    % ---- write "A005_" ----
    telegram(1:5) = uint8('A005_');
    idx = uint8(6);   % next write position (1-based)
    
    % ---- handle NaN/Inf (optional) ----
    x = double(temp);
    if isnan(x) || isinf(x)
        telegram(double(idx):double(idx+2)) = uint8('NaN');
        telegramLen = idx + uint8(2);
        return;
    end
    
    % ---- sign ----
    if x < 0
        telegram(double(idx)) = uint8('-');
        idx = idx + uint8(1);
        x = -x;
    end
    
    % ---- round to 1 decimal: x10 = round(x*10) ----
    x10 = floor(x * 10.0 + 0.5);      % double integer-ish
    ip  = floor(x10 / 10.0);          % integer part (double)
    fp  = x10 - ip * 10.0;            % fractional digit 0..9 (double)
    
    % ---- integer digits -> ASCII (stored reversed) ----
    tmpDigits = zeros(1,10,'uint8');
    dlen = uint8(0);
    
    if ip == 0
        dlen = uint8(1);
        tmpDigits(1) = uint8('0');
    else
        while ip > 0 && dlen < uint8(10)
            dlen = dlen + uint8(1);
            digit = uint8(mod(ip, 10.0));                 % 0..9
            tmpDigits(double(dlen)) = uint8('0') + digit; % ASCII
            ip = floor(ip / 10.0);
        end
    end
    
    % ---- write digits in correct order ----
    k = dlen;
    while k >= uint8(1)
        telegram(double(idx)) = tmpDigits(double(k));
        idx = idx + uint8(1);
        if k == uint8(1)
            break;
        end
        k = k - uint8(1);
    end
    
    % ---- dot + 1 fractional digit ----
    telegram(double(idx)) = uint8('.'); idx = idx + uint8(1);
    telegram(double(idx)) = uint8('0') + uint8(fp); idx = idx + uint8(1);
    
    telegramLen = idx - uint8(1);
end

== matlab function dSpaceModel_2/RS485/MATLAB Function ==
  data: setpoint input double size=1; y output uint8 size=[1, 2]
function y = fcn(setpoint)
    soll = setpoint * (16384 / 100); 
    pcd2 = typecast(int16(soll),'uint8');
y = pcd2;
